simulink model "usb01deneme_hazin"  (R2023a)
settings: Solver=ode5  StartTime=0.0  StopTime=inf  RelTol=1e-3
InitFcn:
  | usbsetup
values from neighbouring files (symbols this model uses):
  K = 1    [usbsetup.m]
  T = Ts    (= 0.01)    [usbsetup.m]
  Td = 0.01    [usbsetup.m]
  Ti = 1    [usbsetup.m]
  Ts_rec = 0.5e-3    (= 0.0005)    [usbsetup.m]
  Ts_send = 0.5e-3    (= 0.0005)    [usbsetup.m]
undefined symbols (not defined in the file or in its folder): Dz, Kd, Serial_Port, Standard_Devices, z0, zp
libraries: sldrtlib x18, dsparch4 x9, slpidlib x1
settings Model: SimulationMode=external  Creator=halil  LastModifiedBy=halil
settings DataIOCC: ReturnWorkspaceOutputs=off
settings DebuggingCC: ParameterPrecisionLossMsg=none
settings HardwareCC: ProdBitPerLong=64  ProdHWDeviceType=Intel->x86-64 (Linux 64)
settings RTWCC: Description=Simulink Desktop Real-Time  SystemTargetFile=sldrt.tlc  TemplateMakefile=sldrt.tmf  RTWCompilerOptimization=on
settings CodeAppCC: MaxIdLength=95
settings SimulinkDesktopRealTimeCC: TargetLibSuffix=_sldrt.a  TargetPreCompLibLocation=C:\Program Files\MATLAB\R2023a\toolbox\sldrt\lib\win64

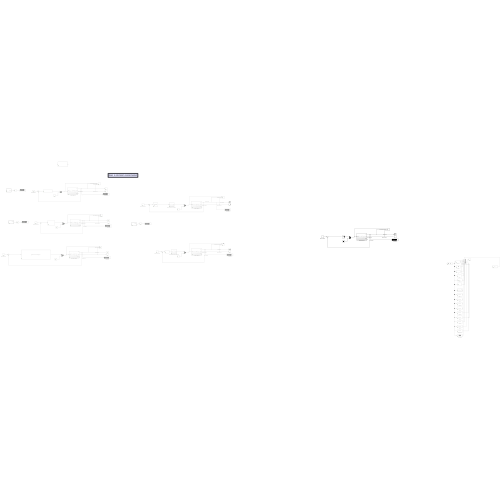
[thumbnail: Simulink's stored preview of the top-level diagram]
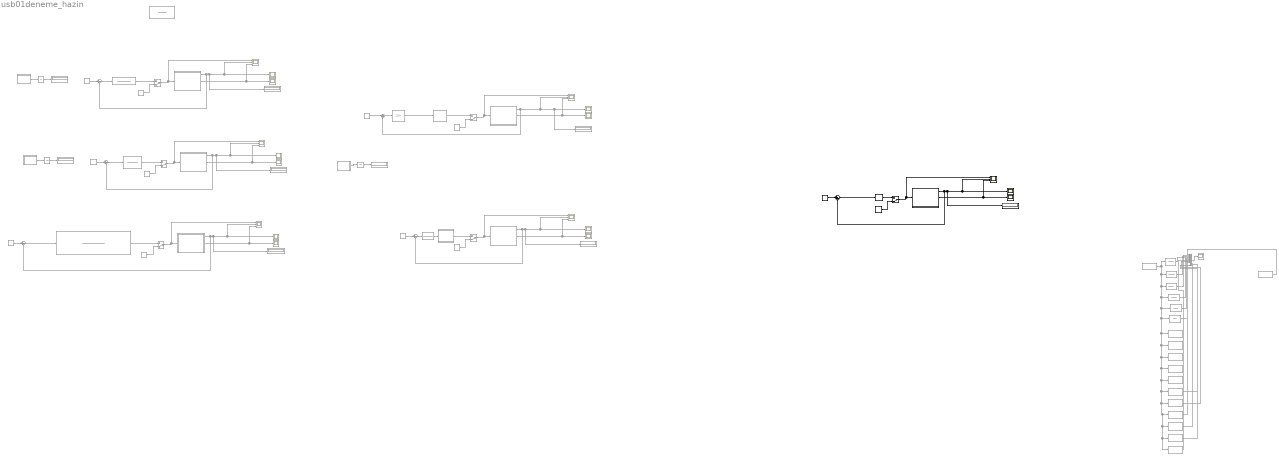
== system usb01deneme_hazin ==
  note: Bazı z-domain çalışmaları
  100fc : TransferFcn  Commented=on  Numerator=[100 0]  Denominator=[1 100]
  1fc : TransferFcn  Commented=on  Numerator=[1 0]  Denominator=[1 1]
  25fc : TransferFcn  Commented=on  Numerator=[25 0]  Denominator=[1 25]
  50fc : TransferFcn  Commented=on  Numerator=[50 0]  Denominator=[1 50]
  5fc : TransferFcn  Commented=on  Numerator=[5 0]  Denominator=[1 5]
  75fc : TransferFcn  Commented=on  Numerator=[75 0]  Denominator=[1 75]
  Angle(deg) : Display
  Angle(deg){1..4,6} (5 alike) : Display  Commented=on
  BugüzelMi? : dsparch4/Biquad Filter  Tag=BlockMethodSubSystem  Commented=on  FilterSource=Dialog parameters  CoeffSource=Specify via dialog  FilterObject=BQF  IIRFiltStruct=Direct form II  BiQuadCoeffs=[1 -1 0 1 -0.999373367998741768 0]  ScaleValues=[0.999686683999370884;1]  IC=0  ICnum=0  ICden=0  a0Flag=Warning  optimizeScaleValues=on  ScaleValueMode=Specify via input port (g)  InputProcessing=Columns as channels (frame based)  roundingMode=Floor  overflowMode=off  scaleValueFracLength=14  denProdOutputFracLength=30  denAccumFracLength=30  secondMemoryFracLength=15
  Constant : Constant  Value=0
  Constant{1..4,6} (5 alike) : Constant  Commented=on  Value=0
  DC Motor Sistemi : Subsystem
  DC Motor Sistemi1 : Subsystem  Commented=on
  DC Motor Sistemi2 : Subsystem  Commented=on
  DC Motor Sistemi3 : Subsystem  Commented=on
  DC Motor Sistemi4 : Subsystem  Commented=on
  DC Motor Sistemi6 : Subsystem  Commented=on
  Data Type Conversion : DataTypeConversion  Commented=on  OutDataTypeStr=double  SaturateOnIntegerOverflow=off  RndMeth=Floor
  Data Type Conversion1 : DataTypeConversion  Commented=on  OutDataTypeStr=double  SaturateOnIntegerOverflow=off  RndMeth=Floor
  Discrete Transfer Fcn : DiscreteTransferFcn  Commented=on  Numerator=[2 -0.2]  Denominator=[1 (1-0.2)]
  Discrete Transfer Fcn1 : DiscreteTransferFcn  Commented=on  Numerator=[(Kd) (-Kd*z0)]  Denominator=[1 (-zp)]  SampleTime=T
  Discrete Transfer Fcn2 : DiscreteTransferFcn  Commented=on  Numerator=[37.5 -37.2]  Denominator=[1 -0.7]  SampleTime=T
  Discrete Transfer Fcn4 : DiscreteTransferFcn  Commented=on  Numerator=[Dz.numerator{1,1}]  Denominator=[Dz.denominator{1,1}]  SampleTime=T
  Display : Display  Commented=on
  Display1 : Display  Commented=on
  Display2 : Display  Commented=on
  Filter : dsparch4/Biquad Filter  Tag=BlockMethodSubSystem  Commented=on  FilterSource=Dialog parameters  CoeffSource=Specify via dialog  FilterObject=BQF  IIRFiltStruct=Direct form II  BiQuadCoeffs=[1 -2 1 1 1.63889042744449531 0.78299941352519975;1 -2 1 1 1.39413928992720804 0.516727106758841592;1 -1 0 1 0.659452728771293573 0]  ScaleValues=[0.0360272465201760816;0.0306469542079083335;0.170273635614353186;1]  IC=0  ICnum=0  ICden=0  a0Flag=Warning  optimizeScaleValues=on  ScaleValueMode=Specify via input port (g)  InputProcessing=Columns as channels (frame based)  roundingMode=Floor  overflowMode=off  scaleValueFracLength=14  denProdOutputFracLength=30  denAccumFracLength=30  secondMemoryFracLength=15
  Filter1 : dsparch4/Biquad Filter  Tag=BlockMethodSubSystem  Commented=on  FilterSource=Dialog parameters  CoeffSource=Specify via dialog  FilterObject=BQF  IIRFiltStruct=Direct form II  BiQuadCoeffs=[1 -2 1 1 -0.751668315831577671 0.502252814025592853;1 -2 1 1 -0.555983969636365316 0.111166275533815195]  ScaleValues=[0.563480282464292603;0.416787561292545128;1]  IC=0  ICnum=0  ICden=0  a0Flag=Warning  optimizeScaleValues=on  ScaleValueMode=Specify via input port (g)  InputProcessing=Columns as channels (frame based)  roundingMode=Floor  overflowMode=off  scaleValueFracLength=14  denProdOutputFracLength=30  denAccumFracLength=30  secondMemoryFracLength=15
  Filter2 : dsparch4/Biquad Filter  Tag=BlockMethodSubSystem  Commented=on  FilterSource=Dialog parameters  CoeffSource=Specify via dialog  FilterObject=BQF  IIRFiltStruct=Direct form II  BiQuadCoeffs=[1 -2 1 1 -1.7220160678191494 0.756195048099618239]  ScaleValues=[0.869552778979691854;1]  IC=0  ICnum=0  ICden=0  a0Flag=Warning  optimizeScaleValues=on  ScaleValueMode=Specify via input port (g)  InputProcessing=Columns as channels (frame based)  roundingMode=Floor  overflowMode=off  scaleValueFracLength=14  denProdOutputFracLength=30  denAccumFracLength=30  secondMemoryFracLength=15
  Filter3 : dsparch4/Biquad Filter  Tag=BlockMethodSubSystem  Commented=on  FilterSource=Dialog parameters  CoeffSource=Specify via dialog  FilterObject=BQF  IIRFiltStruct=Direct form II  BiQuadCoeffs=[1 -2 1 1 -1.97197387617265707 0.972361217649310716]  ScaleValues=[0.986083773455491919;1]  IC=0  ICnum=0  ICden=0  a0Flag=Warning  optimizeScaleValues=on  ScaleValueMode=Specify via input port (g)  InputProcessing=Columns as channels (frame based)  roundingMode=Floor  overflowMode=off  scaleValueFracLength=14  denProdOutputFracLength=30  denAccumFracLength=30  secondMemoryFracLength=15
  Filter4 : dsparch4/Biquad Filter  Tag=BlockMethodSubSystem  Commented=on  FilterSource=Dialog parameters  CoeffSource=Specify via dialog  FilterObject=BQF  IIRFiltStruct=Direct form II  BiQuadCoeffs=[1 -1 0 1 -0.993767790272316875 0]  ScaleValues=[0.996883895136158382;1]  IC=0  ICnum=0  ICden=0  a0Flag=Warning  optimizeScaleValues=on  ScaleValueMode=Specify via input port (g)  InputProcessing=Columns as channels (frame based)  roundingMode=Floor  overflowMode=off  scaleValueFracLength=14  denProdOutputFracLength=30  denAccumFracLength=30  secondMemoryFracLength=15
  Filter5 : dsparch4/Biquad Filter  Tag=BlockMethodSubSystem  Commented=on  FilterSource=Dialog parameters  CoeffSource=Specify via dialog  FilterObject=BQF  IIRFiltStruct=Direct form II  BiQuadCoeffs=[1 -1 0 1 -0.981326377391473437 0]  ScaleValues=[0.990663188695736663;1]  IC=0  ICnum=0  ICden=0  a0Flag=Warning  optimizeScaleValues=on  ScaleValueMode=Specify via input port (g)  InputProcessing=Columns as channels (frame based)  roundingMode=Floor  overflowMode=off  scaleValueFracLength=14  denProdOutputFracLength=30  denAccumFracLength=30  secondMemoryFracLength=15
  Filter6 : dsparch4/Biquad Filter  Tag=BlockMethodSubSystem  Commented=on  FilterSource=Dialog parameters  CoeffSource=Specify via dialog  FilterObject=BQF  IIRFiltStruct=Direct form II  BiQuadCoeffs=[1 -1 0 1 -0.998456046873542391 0]  ScaleValues=[0.999228023436771196;1]  IC=0  ICnum=0  ICden=0  a0Flag=Warning  optimizeScaleValues=on  ScaleValueMode=Specify via input port (g)  InputProcessing=Columns as channels (frame based)  roundingMode=Floor  overflowMode=off  scaleValueFracLength=14  denProdOutputFracLength=30  denAccumFracLength=30  secondMemoryFracLength=15
  Filter7 : dsparch4/Biquad Filter  Tag=BlockMethodSubSystem  Commented=on  FilterSource=Dialog parameters  CoeffSource=Specify via dialog  FilterObject=BQF  IIRFiltStruct=Direct form II  BiQuadCoeffs=[1 -1 0 1 -0.999227725423996294 0]  ScaleValues=[0.999613862711998147;1]  IC=0  ICnum=0  ICden=0  a0Flag=Warning  optimizeScaleValues=on  ScaleValueMode=Specify via input port (g)  InputProcessing=Columns as channels (frame based)  roundingMode=Floor  overflowMode=off  scaleValueFracLength=14  denProdOutputFracLength=30  denAccumFracLength=30  secondMemoryFracLength=15
  Integrator : Integrator  Commented=on
  Integrator1 : Integrator  Commented=on
  Integrator2 : Integrator  Commented=on
  MATLAB Function : MATLAB Function  Commented=on  TreatAsAtomicUnit=on
  MATLAB Function1 : MATLAB Function  Commented=on  TreatAsAtomicUnit=on
  MATLAB Function2 : MATLAB Function  Commented=on  TreatAsAtomicUnit=on
  Manual Switch : ManualSwitch  CurrentSetting=0
  Manual Switch{1..4,6} (5 alike) : ManualSwitch  Commented=on  CurrentSetting=0
  Mux : Mux  Commented=on  Inputs=13
  PID Controller1 : slpidlib/PID Controller  Controller=PID  Form=Ideal  TimeDomain=Continuous-time  UseExternalTs=off  SampleTime=-1  IntegratorMethod=Forward Euler  FilterMethod=Forward Euler  ControllerParametersSource=internal  P=1  I=1  UseKiTs=off  D=0.01  N=100  UseFilter=on  TunerSelectOption=Transfer Function Based (PID Tuner App)  InitialConditionSource=internal  InitialConditionForIntegrator=0  InitialConditionForFilter=0  DifferentiatorICPrevScaledInput=0  ExternalReset=none  TrackingMode=off  Kt=1  LimitOutput=on  SatLimitsSource=internal  UpperSaturationLimit=6  LowerSaturationLimit=-6  LinearizeAsGain=off  AntiWindupMode=none  Kb=1  LimitIntegrator=off  UpperIntegratorSaturationLimit=inf  LowerIntegratorSaturationLimit=-inf  POutMin=[]  POutMax=[]  IOutMin=[]  IOutMax=[]  DOutMin=[]  DOutMax=[]  NOutMin=[]  NOutMax=[]  SumOutMin=[]  SumOutMax=[]  SaturationOutMin=[]  SaturationOutMax=[]  PParamMin=[]  PParamMax=[]  IParamMin=[]  IParamMax=[]  DParamMin=[]  DParamMax=[]  NParamMin=[]  NParamMax=[]  KbParamMin=[]  KbParamMax=[]  KtParamMin=[]  KtParamMax=[]  KbOutMin=[]  KbOutMax=[]  KtOutMin=[]  KtOutMax=[]  IntegratorOutMin=[]  IntegratorOutMax=[]  FilterOutMin=[]  FilterOutMax=[]  SumI1OutMin=[]  SumI1OutMax=[]  SumI2OutMin=[]  SumI2OutMax=[]  SumI3OutMin=[]  SumI3OutMax=[]  SumI4OutMin=[]  SumI4OutMax=[]  SumDOutMin=[]  SumDOutMax=[]  DifferentiatorOutMin=[]  DifferentiatorOutMax=[]  FilterDiffOutCoefMin=[]  FilterDiffOutCoefMax=[]  ReciprocalOutMin=[]  ReciprocalOutMax=[]  SumDenOutMin=[]  SumDenOutMax=[]  SumNumOutMin=[]  SumNumOutMax=[]  DivideOutMin=[]  DivideOutMax=[]  UdiffTsProdOutMin=[]  UdiffTsProdOutMax=[]  NTsProdOutMin=[]  NTsProdOutMax=[]  UintegralTsProdOutMin=[]  UintegralTsProdOutMax=[]  UngainTsProdOutMin=[]  UngainTsProdOutMax=[]  ClampingZeroOutDataTypeStr=Inherit: Inherit via back propagation  ClampingZeroOutMin=[]  ClampingZeroOutMax=[]  FilterDenConstantOutDataTypeStr=Inherit: Inherit via back propagation  FilterDenConstantOutMin=[]  FilterDenConstantOutMax=[]  PCopyOutDataTypeStr=Inherit: Inherit via back propagation  PCopyOutMin=[]  PCopyOutMax=[]  NCopyOutDataTypeStr=Inherit: Inherit via back propagation  NCopyOutMin=[]  NCopyOutMax=[]  IntegratorContinuousStateAttributes=''  IntegratorStateMustResolveToSignalObject=off  IntegratorRTWStateStorageClass=Auto  FilterContinuousStateAttributes=''  FilterStateMustResolveToSignalObject=off  FilterRTWStateStorageClass=Auto  ParallelPVariant=Passthrough  IdealPVariant=InternalParameters  IVariant=InternalParameters  DVariant=InternalParameters  IntegratorVariant=Continuous  SatVariant=Enabled  AWVariant=Passthrough  PCopyVariant=Disabled  TRVariant=Disabled  FdbkBlocksVariant=Forward  IdealPFdbkVariant=Disabled  SatFdbkVariant=Disabled  DerivativeFilterVariant=ContFilter  NVariant=InternalParameters  NCopyVariant=Disabled  FilterICVariant=InternalICsFilter  IntegratorICVariant=InternalICs  ExternalResetVariant=Disabled  TRSumVariant=Passthrough  SumFdbkVariant=Disabled  SumVariant=Sum_PID  TsampFilterVariant=InternalTs  TsampNgainVariant=Passthrough  TsampIntegralVariant=Disabled_SignalSpec  ExternalSaturationOutDataTypeStr=Inherit: Same as second input
  PID(frequence domain emulation) : Subsystem  Commented=on
  PID(time domain emulation) : Subsystem  Commented=on
  Scope{,4,6,8..9,11..12,14..15,20..21} (11 alike) : Scope  Commented=on
  Scope1 : Scope  NumInputPorts=3
  Scope{2,7,10,13,19} (5 alike) : Scope  Commented=on  NumInputPorts=3
  Scope3 : Scope
  Scope5 : Scope
  Sum : Sum  Inputs=|+-
  Sum{1..4,6} (5 alike) : Sum  Commented=on  Inputs=|+-
  Transfer Fcn1 : TransferFcn  Commented=on  Numerator=[90/2.1]  Denominator=[0.2/4 1]
  Zero-Order Hold : ZeroOrderHold  Commented=on  SampleTime=T
  differentiFilter : DiscreteFir  Tag=BlockMethodSubSystem  Commented=on  Coefficients=[0.10162245249798578 0.462115751014000098 -0.462115751014000098 -0.10162245249798578]  InputProcessing=Columns as channels (frame based)
  numericd1 : Subsystem  Tag=BlockMethodSubSystem  Commented=on
  setPoint(degree) : Constant  Value=100
  setPoint(degree)1 : Constant  Commented=on  Value=0
  setPoint(degree)2 : Constant  Commented=on  Value=100
  setPoint(degree)3 : Constant  Commented=on  Value=100
  setPoint(degree)4 : Constant  Commented=on  Value=100
  setPoint(degree)6 : Constant  Commented=on  Value=0
  wires:
  DC Motor Sistemi/1(Açı) -> Sum/2, Scope1/2, Scope3/1, Angle(deg)/1  "Angle(degree)"
  Sum/1 -> PID Controller1/1
  50fc/1 -> Mux/4  "dq"
  Mux/1 -> Scope/1
  Data Type Conversion/1 -> differentiFilter/1, BugüzelMi?/1, Filter7/1, Filter6/1, Filter5/1, Filter4/1, Filter3/1, Filter2/1, Filter1/1, Filter/1, numericd1/1(In), 1fc/1, 5fc/1, 25fc/1, 75fc/1, 100fc/1, 50fc/1
  Constant/1 -> Manual Switch/2
  Manual Switch/1 -> Scope1/1, DC Motor Sistemi/1(Voltaj)  "control signal(u)(Voltage)"
  Data Type Conversion1/1 -> Mux/1
  100fc/1 -> Mux/3
  75fc/1 -> Mux/2
  25fc/1 -> Mux/5
  5fc/1 -> Mux/6
  Filter4/1 -> Mux/13
  Filter5/1 -> Mux/9
  Filter6/1 -> Mux/10
  Filter7/1 -> Mux/11
  BugüzelMi?/1 -> Mux/12
  differentiFilter/1 -> Mux/8
  DC Motor Sistemi/2(Hız) -> Scope1/3, Scope5/1  "filteredSpeed(1/s)"
  1fc/1 -> Mux/7
  PID Controller1/1 -> Manual Switch/1
  setPoint(degree)/1 -> Sum/1
  Manual Switch1/1 -> Scope2/1, DC Motor Sistemi1/1(Voltaj)  "control signal(u)(Voltage)"
  DC Motor Sistemi1/2(Hız) -> Scope2/3, Scope6/1  "filteredSpeed(1/s)"
  PID(time domain emulation)/1(u[k]) -> Manual Switch1/1
  Constant1/1 -> Manual Switch1/2
  DC Motor Sistemi1/1(Açı) -> Scope2/2, Angle(deg)1/1, Scope4/1, Sum1/2  "Angle(degree)"
  setPoint(degree)1/1 -> Sum1/1
  Sum1/1 -> Zero-Order Hold/1
  Zero-Order Hold/1 -> PID(time domain emulation)/1(e[k])
  setPoint(degree)2/1 -> Sum3/1
  Manual Switch2/1 -> Scope7/1, DC Motor Sistemi2/1(Voltaj)  "control signal(u)(Voltage)"
  DC Motor Sistemi2/2(Hız) -> Scope7/3, Scope9/1  "filteredSpeed(1/s)"
  PID(frequence domain emulation)/1(u(t)) -> Manual Switch2/1
  Constant2/1 -> Manual Switch2/2
  DC Motor Sistemi2/1(Açı) -> Sum3/2, Scope7/2, Scope8/1, Angle(deg)2/1  "Angle(degree)"
  Discrete Transfer Fcn/1 -> PID(frequence domain emulation)/1(e(t))
  Sum3/1 -> Discrete Transfer Fcn/1
  DC Motor Sistemi3/2(Hız) -> Scope10/3, Scope12/1  "filteredSpeed(1/s)"
  Constant3/1 -> Manual Switch3/2
  DC Motor Sistemi3/1(Açı) -> Sum2/2, Scope10/2, Scope11/1, Angle(deg)3/1  "Angle(degree)"
  setPoint(degree)3/1 -> Sum2/1
  Manual Switch3/1 -> Scope10/1, DC Motor Sistemi3/1(Voltaj)  "control signal(u)(Voltage)"
  Sum2/1 -> Discrete Transfer Fcn1/1
  Discrete Transfer Fcn1/1 -> Manual Switch3/1
  MATLAB Function/1(norme) -> Integrator/1
  Integrator/1 -> Display/1
  Integrator1/1 -> Display1/1
  MATLAB Function1/1(norme) -> Integrator1/1
  Constant4/1 -> Manual Switch4/2
  DC Motor Sistemi4/2(Hız) -> Scope13/3, Scope15/1  "filteredSpeed(1/s)"
  Manual Switch4/1 -> Scope13/1, DC Motor Sistemi4/1(Voltaj)  "control signal(u)(Voltage)"
  DC Motor Sistemi4/1(Açı) -> Sum4/2, Scope13/2, Scope14/1, Angle(deg)4/1  "Angle(degree)"
  Discrete Transfer Fcn2/1 -> Manual Switch4/1
  setPoint(degree)4/1 -> Sum4/1
  Sum4/1 -> Discrete Transfer Fcn2/1
  MATLAB Function2/1(norme) -> Integrator2/1
  Integrator2/1 -> Display2/1
  Sum6/1 -> Discrete Transfer Fcn4/1
  setPoint(degree)6/1 -> Sum6/1
  Discrete Transfer Fcn4/1 -> Manual Switch6/1
  Manual Switch6/1 -> Scope19/1, DC Motor Sistemi6/1(Voltaj)  "control signal(u)(Voltage)"
  Constant6/1 -> Manual Switch6/2
  DC Motor Sistemi6/2(Hız) -> Scope19/3, Scope21/1  "filteredSpeed(1/s)"
  DC Motor Sistemi6/1(Açı) -> Sum6/2, Scope19/2, Scope20/1, Angle(deg)6/1  "Angle(degree)"

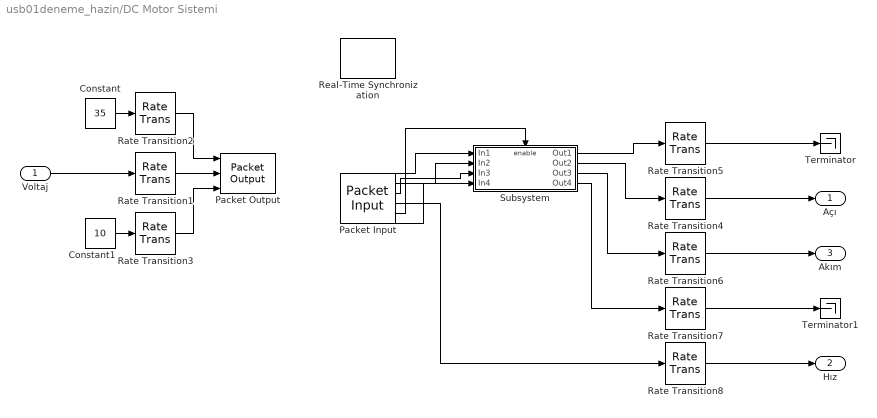
== system usb01deneme_hazin/DC Motor Sistemi ==
  Voltaj : Inport
  Constant : Constant  Value=35
  Constant1 : Constant  Value=10
  Packet Input : sldrtlib/Packet Input  SampleTime=Ts_rec  MaxMissedTicks=1000  ShowMissedTicks=off  YieldWhenWaiting=off  DrvName=Standard_Devices/Serial_Port  DrvAddress=4  DrvOptions=[9600 8 0 0 0 0 0 0]  PacketSize=14  DataTypes={'uint8','single','single','single','uint8'}  ShowReady=on  ShowError=off  PacketID=1  ByteOrder=1  ShowTimestamp=off
      settings: AttributesFormatString=Serial Port [4]
  Packet Output : sldrtlib/Packet Output  SampleTime=Ts_send  MaxMissedTicks=1000  ShowMissedTicks=off  YieldWhenWaiting=off  DrvName=Standard_Devices/Serial_Port  DrvAddress=4  DrvOptions=[9600 8 0 0 0 0 0 0]  PacketSize=6  DataTypes={'uint8','single','uint8'}  ShowReady=off  ShowError=off  PacketID=1  ByteOrder=1  InitialValue=[]  FinalValue=[]
      settings: AttributesFormatString=Serial Port [4]
  Rate Transition1 : RateTransition  OutPortSampleTime=Ts_send
  Rate Transition2 : RateTransition  OutPortSampleTime=Ts_send
  Rate Transition3 : RateTransition  OutPortSampleTime=Ts_send
  Rate Transition{4..8} (5 alike) : RateTransition  OutPortSampleTime=Ts_algo
  Real-Time Synchronization : sldrtlib/Real-Time Synchronization  SampleTime=Ts_rec  MaxMissedTicks=1000  ShowMissedTicks=off  YieldWhenWaiting=off
  Subsystem : Subsystem
  Terminator : Terminator
  Terminator1 : Terminator
  Açı : Outport
  Hız : Outport  Port=2
  Akım : Outport  Port=3
  wires:
  Rate Transition3/1 -> Packet Output/3
  Rate Transition1/1 -> Packet Output/2
  Subsystem/1(Out1) -> Rate Transition5/1
  Packet Input/2 -> Subsystem/2(In2)
  Rate Transition2/1 -> Packet Output/1
  Packet Input/3 -> Subsystem/3(In3)
  Subsystem/3(Out3) -> Rate Transition6/1
  Subsystem/4(Out4) -> Rate Transition7/1
  Packet Input/1 -> Subsystem/1(In1)
  Packet Input/5 -> Subsystem/Enable
  Subsystem/2(Out2) -> Rate Transition4/1
  Rate Transition4/1 -> Açı/1
  Voltaj/1 -> Rate Transition1/1
  Constant/1 -> Rate Transition2/1
  Rate Transition7/1 -> Terminator1/1
  Constant1/1 -> Rate Transition3/1
  Rate Transition5/1 -> Terminator/1
  Packet Input/4 -> Rate Transition8/1
  Rate Transition8/1 -> Hız/1
  Packet Input/6 -> Subsystem/4(In4)
  Rate Transition6/1 -> Akım/1

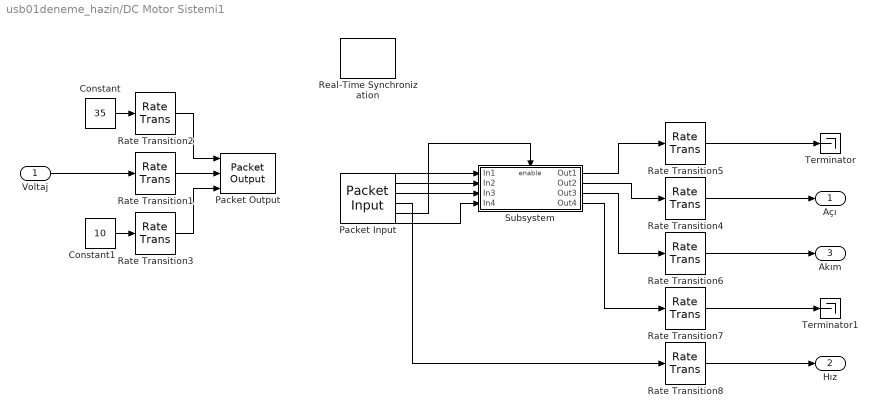
== system usb01deneme_hazin/DC Motor Sistemi1 ==
  Voltaj : Inport
  Constant : Constant  Value=35
  Constant1 : Constant  Value=10
  Packet Input : sldrtlib/Packet Input  SampleTime=Ts_rec  MaxMissedTicks=1000  ShowMissedTicks=off  YieldWhenWaiting=off  DrvName=Standard_Devices/Serial_Port  DrvAddress=4  DrvOptions=[9600 8 0 0 0 0 0 0]  PacketSize=14  DataTypes={'uint8','single','single','single','uint8'}  ShowReady=on  ShowError=off  PacketID=1  ByteOrder=1  ShowTimestamp=off
      settings: AttributesFormatString=Serial Port [4]
  Packet Output : sldrtlib/Packet Output  SampleTime=Ts_send  MaxMissedTicks=1000  ShowMissedTicks=off  YieldWhenWaiting=off  DrvName=Standard_Devices/Serial_Port  DrvAddress=4  DrvOptions=[9600 8 0 0 0 0 0 0]  PacketSize=6  DataTypes={'uint8','single','uint8'}  ShowReady=off  ShowError=off  PacketID=1  ByteOrder=1  InitialValue=[]  FinalValue=[]
      settings: AttributesFormatString=Serial Port [4]
  Rate Transition1 : RateTransition  OutPortSampleTime=Ts_send
  Rate Transition2 : RateTransition  OutPortSampleTime=Ts_send
  Rate Transition3 : RateTransition  OutPortSampleTime=Ts_send
  Rate Transition{4..8} (5 alike) : RateTransition  OutPortSampleTime=Ts_algo
  Real-Time Synchronization : sldrtlib/Real-Time Synchronization  SampleTime=Ts_rec  MaxMissedTicks=1000  ShowMissedTicks=off  YieldWhenWaiting=off
  Subsystem : Subsystem
  Terminator : Terminator
  Terminator1 : Terminator
  Açı : Outport
  Hız : Outport  Port=2
  Akım : Outport  Port=3
  wires:
  Rate Transition3/1 -> Packet Output/3
  Rate Transition1/1 -> Packet Output/2
  Subsystem/1(Out1) -> Rate Transition5/1
  Packet Input/2 -> Subsystem/2(In2)
  Rate Transition2/1 -> Packet Output/1
  Packet Input/3 -> Subsystem/3(In3)
  Subsystem/3(Out3) -> Rate Transition6/1
  Subsystem/4(Out4) -> Rate Transition7/1
  Packet Input/1 -> Subsystem/1(In1)
  Packet Input/5 -> Subsystem/Enable
  Subsystem/2(Out2) -> Rate Transition4/1
  Rate Transition4/1 -> Açı/1
  Voltaj/1 -> Rate Transition1/1
  Constant/1 -> Rate Transition2/1
  Rate Transition7/1 -> Terminator1/1
  Constant1/1 -> Rate Transition3/1
  Rate Transition5/1 -> Terminator/1
  Packet Input/4 -> Rate Transition8/1
  Rate Transition8/1 -> Hız/1
  Packet Input/6 -> Subsystem/4(In4)
  Rate Transition6/1 -> Akım/1

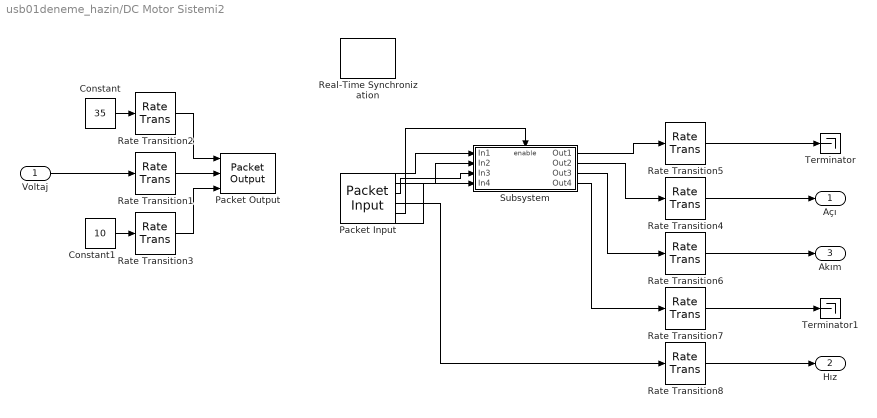
== system usb01deneme_hazin/DC Motor Sistemi2 ==
  Voltaj : Inport
  Constant : Constant  Value=35
  Constant1 : Constant  Value=10
  Packet Input : sldrtlib/Packet Input  SampleTime=Ts_rec  MaxMissedTicks=1000  ShowMissedTicks=off  YieldWhenWaiting=off  DrvName=Standard_Devices/Serial_Port  DrvAddress=4  DrvOptions=[9600 8 0 0 0 0 0 0]  PacketSize=14  DataTypes={'uint8','single','single','single','uint8'}  ShowReady=on  ShowError=off  PacketID=1  ByteOrder=1  ShowTimestamp=off
      settings: AttributesFormatString=Serial Port [4]
  Packet Output : sldrtlib/Packet Output  SampleTime=Ts_send  MaxMissedTicks=1000  ShowMissedTicks=off  YieldWhenWaiting=off  DrvName=Standard_Devices/Serial_Port  DrvAddress=4  DrvOptions=[9600 8 0 0 0 0 0 0]  PacketSize=6  DataTypes={'uint8','single','uint8'}  ShowReady=off  ShowError=off  PacketID=1  ByteOrder=1  InitialValue=[]  FinalValue=[]
      settings: AttributesFormatString=Serial Port [4]
  Rate Transition1 : RateTransition  OutPortSampleTime=Ts_send
  Rate Transition2 : RateTransition  OutPortSampleTime=Ts_send
  Rate Transition3 : RateTransition  OutPortSampleTime=Ts_send
  Rate Transition{4..8} (5 alike) : RateTransition  OutPortSampleTime=Ts_algo
  Real-Time Synchronization : sldrtlib/Real-Time Synchronization  SampleTime=Ts_rec  MaxMissedTicks=1000  ShowMissedTicks=off  YieldWhenWaiting=off
  Subsystem : Subsystem
  Terminator : Terminator
  Terminator1 : Terminator
  Açı : Outport
  Hız : Outport  Port=2
  Akım : Outport  Port=3
  wires:
  Rate Transition3/1 -> Packet Output/3
  Rate Transition1/1 -> Packet Output/2
  Subsystem/1(Out1) -> Rate Transition5/1
  Packet Input/2 -> Subsystem/2(In2)
  Rate Transition2/1 -> Packet Output/1
  Packet Input/3 -> Subsystem/3(In3)
  Subsystem/3(Out3) -> Rate Transition6/1
  Subsystem/4(Out4) -> Rate Transition7/1
  Packet Input/1 -> Subsystem/1(In1)
  Packet Input/5 -> Subsystem/Enable
  Subsystem/2(Out2) -> Rate Transition4/1
  Rate Transition4/1 -> Açı/1
  Voltaj/1 -> Rate Transition1/1
  Constant/1 -> Rate Transition2/1
  Rate Transition7/1 -> Terminator1/1
  Constant1/1 -> Rate Transition3/1
  Rate Transition5/1 -> Terminator/1
  Packet Input/4 -> Rate Transition8/1
  Rate Transition8/1 -> Hız/1
  Packet Input/6 -> Subsystem/4(In4)
  Rate Transition6/1 -> Akım/1

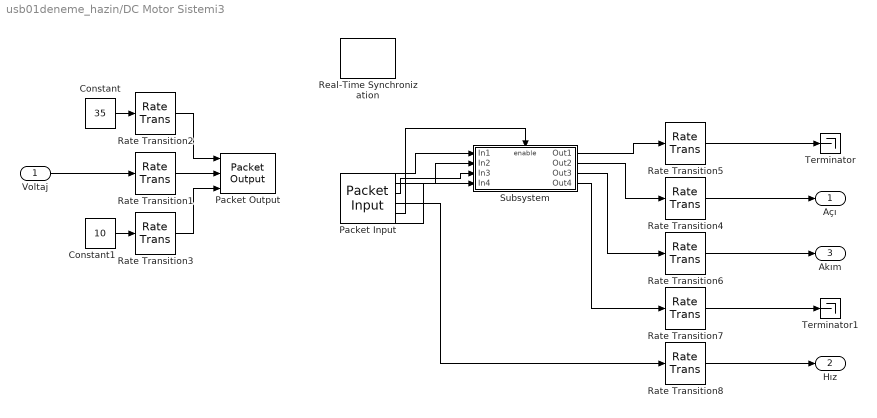
== system usb01deneme_hazin/DC Motor Sistemi3 ==
  Voltaj : Inport
  Constant : Constant  Value=35
  Constant1 : Constant  Value=10
  Packet Input : sldrtlib/Packet Input  SampleTime=Ts_rec  MaxMissedTicks=1000  ShowMissedTicks=off  YieldWhenWaiting=off  DrvName=Standard_Devices/Serial_Port  DrvAddress=4  DrvOptions=[9600 8 0 0 0 0 0 0]  PacketSize=14  DataTypes={'uint8','single','single','single','uint8'}  ShowReady=on  ShowError=off  PacketID=1  ByteOrder=1  ShowTimestamp=off
      settings: AttributesFormatString=Serial Port [4]
  Packet Output : sldrtlib/Packet Output  SampleTime=Ts_send  MaxMissedTicks=1000  ShowMissedTicks=off  YieldWhenWaiting=off  DrvName=Standard_Devices/Serial_Port  DrvAddress=4  DrvOptions=[9600 8 0 0 0 0 0 0]  PacketSize=6  DataTypes={'uint8','single','uint8'}  ShowReady=off  ShowError=off  PacketID=1  ByteOrder=1  InitialValue=[]  FinalValue=[]
      settings: AttributesFormatString=Serial Port [4]
  Rate Transition1 : RateTransition  OutPortSampleTime=Ts_send
  Rate Transition2 : RateTransition  OutPortSampleTime=Ts_send
  Rate Transition3 : RateTransition  OutPortSampleTime=Ts_send
  Rate Transition{4..8} (5 alike) : RateTransition  OutPortSampleTime=Ts_algo
  Real-Time Synchronization : sldrtlib/Real-Time Synchronization  SampleTime=Ts_rec  MaxMissedTicks=1000  ShowMissedTicks=off  YieldWhenWaiting=off
  Subsystem : Subsystem
  Terminator : Terminator
  Terminator1 : Terminator
  Açı : Outport
  Hız : Outport  Port=2
  Akım : Outport  Port=3
  wires:
  Rate Transition3/1 -> Packet Output/3
  Rate Transition1/1 -> Packet Output/2
  Subsystem/1(Out1) -> Rate Transition5/1
  Packet Input/2 -> Subsystem/2(In2)
  Rate Transition2/1 -> Packet Output/1
  Packet Input/3 -> Subsystem/3(In3)
  Subsystem/3(Out3) -> Rate Transition6/1
  Subsystem/4(Out4) -> Rate Transition7/1
  Packet Input/1 -> Subsystem/1(In1)
  Packet Input/5 -> Subsystem/Enable
  Subsystem/2(Out2) -> Rate Transition4/1
  Rate Transition4/1 -> Açı/1
  Voltaj/1 -> Rate Transition1/1
  Constant/1 -> Rate Transition2/1
  Rate Transition7/1 -> Terminator1/1
  Constant1/1 -> Rate Transition3/1
  Rate Transition5/1 -> Terminator/1
  Packet Input/4 -> Rate Transition8/1
  Rate Transition8/1 -> Hız/1
  Packet Input/6 -> Subsystem/4(In4)
  Rate Transition6/1 -> Akım/1

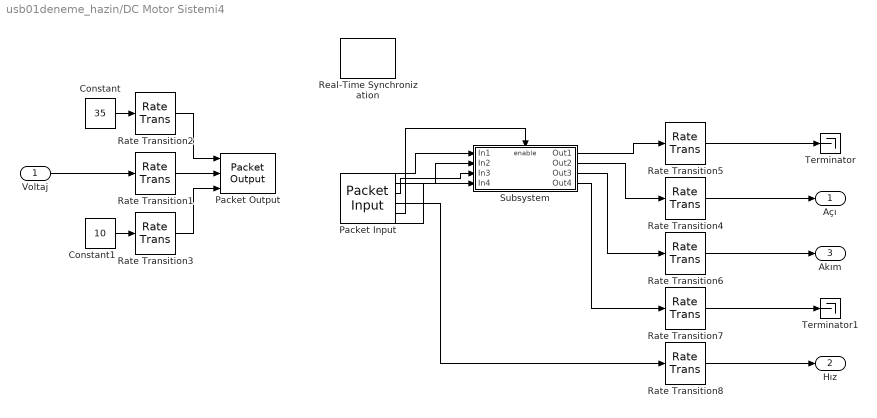
== system usb01deneme_hazin/DC Motor Sistemi4 ==
  Voltaj : Inport
  Constant : Constant  Value=35
  Constant1 : Constant  Value=10
  Packet Input : sldrtlib/Packet Input  SampleTime=Ts_rec  MaxMissedTicks=1000  ShowMissedTicks=off  YieldWhenWaiting=off  DrvName=Standard_Devices/Serial_Port  DrvAddress=4  DrvOptions=[9600 8 0 0 0 0 0 0]  PacketSize=14  DataTypes={'uint8','single','single','single','uint8'}  ShowReady=on  ShowError=off  PacketID=1  ByteOrder=1  ShowTimestamp=off
      settings: AttributesFormatString=Serial Port [4]
  Packet Output : sldrtlib/Packet Output  SampleTime=Ts_send  MaxMissedTicks=1000  ShowMissedTicks=off  YieldWhenWaiting=off  DrvName=Standard_Devices/Serial_Port  DrvAddress=4  DrvOptions=[9600 8 0 0 0 0 0 0]  PacketSize=6  DataTypes={'uint8','single','uint8'}  ShowReady=off  ShowError=off  PacketID=1  ByteOrder=1  InitialValue=[]  FinalValue=[]
      settings: AttributesFormatString=Serial Port [4]
  Rate Transition1 : RateTransition  OutPortSampleTime=Ts_send
  Rate Transition2 : RateTransition  OutPortSampleTime=Ts_send
  Rate Transition3 : RateTransition  OutPortSampleTime=Ts_send
  Rate Transition{4..8} (5 alike) : RateTransition  OutPortSampleTime=Ts_algo
  Real-Time Synchronization : sldrtlib/Real-Time Synchronization  SampleTime=Ts_rec  MaxMissedTicks=1000  ShowMissedTicks=off  YieldWhenWaiting=off
  Subsystem : Subsystem
  Terminator : Terminator
  Terminator1 : Terminator
  Açı : Outport
  Hız : Outport  Port=2
  Akım : Outport  Port=3
  wires:
  Rate Transition3/1 -> Packet Output/3
  Rate Transition1/1 -> Packet Output/2
  Subsystem/1(Out1) -> Rate Transition5/1
  Packet Input/2 -> Subsystem/2(In2)
  Rate Transition2/1 -> Packet Output/1
  Packet Input/3 -> Subsystem/3(In3)
  Subsystem/3(Out3) -> Rate Transition6/1
  Subsystem/4(Out4) -> Rate Transition7/1
  Packet Input/1 -> Subsystem/1(In1)
  Packet Input/5 -> Subsystem/Enable
  Subsystem/2(Out2) -> Rate Transition4/1
  Rate Transition4/1 -> Açı/1
  Voltaj/1 -> Rate Transition1/1
  Constant/1 -> Rate Transition2/1
  Rate Transition7/1 -> Terminator1/1
  Constant1/1 -> Rate Transition3/1
  Rate Transition5/1 -> Terminator/1
  Packet Input/4 -> Rate Transition8/1
  Rate Transition8/1 -> Hız/1
  Packet Input/6 -> Subsystem/4(In4)
  Rate Transition6/1 -> Akım/1

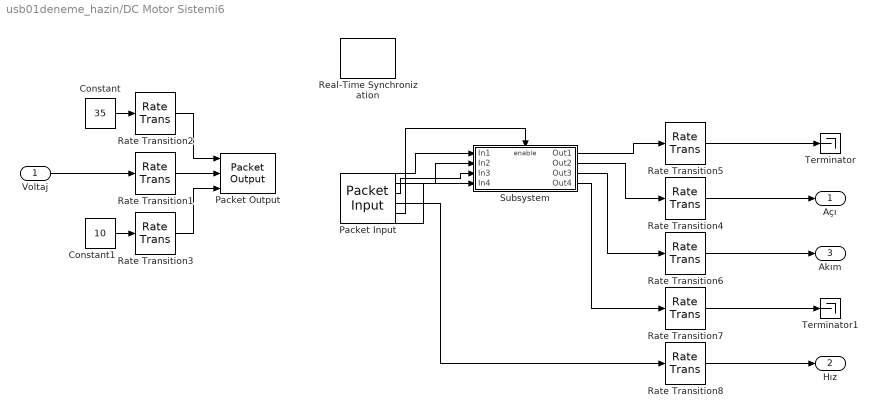
== system usb01deneme_hazin/DC Motor Sistemi6 ==
  Voltaj : Inport
  Constant : Constant  Value=35
  Constant1 : Constant  Value=10
  Packet Input : sldrtlib/Packet Input  SampleTime=Ts_rec  MaxMissedTicks=1000  ShowMissedTicks=off  YieldWhenWaiting=off  DrvName=Standard_Devices/Serial_Port  DrvAddress=4  DrvOptions=[9600 8 0 0 0 0 0 0]  PacketSize=14  DataTypes={'uint8','single','single','single','uint8'}  ShowReady=on  ShowError=off  PacketID=1  ByteOrder=1  ShowTimestamp=off
      settings: AttributesFormatString=Serial Port [4]
  Packet Output : sldrtlib/Packet Output  SampleTime=Ts_send  MaxMissedTicks=1000  ShowMissedTicks=off  YieldWhenWaiting=off  DrvName=Standard_Devices/Serial_Port  DrvAddress=4  DrvOptions=[9600 8 0 0 0 0 0 0]  PacketSize=6  DataTypes={'uint8','single','uint8'}  ShowReady=off  ShowError=off  PacketID=1  ByteOrder=1  InitialValue=[]  FinalValue=[]
      settings: AttributesFormatString=Serial Port [4]
  Rate Transition1 : RateTransition  OutPortSampleTime=Ts_send
  Rate Transition2 : RateTransition  OutPortSampleTime=Ts_send
  Rate Transition3 : RateTransition  OutPortSampleTime=Ts_send
  Rate Transition{4..8} (5 alike) : RateTransition  OutPortSampleTime=Ts_algo
  Real-Time Synchronization : sldrtlib/Real-Time Synchronization  SampleTime=Ts_rec  MaxMissedTicks=1000  ShowMissedTicks=off  YieldWhenWaiting=off
  Subsystem : Subsystem
  Terminator : Terminator
  Terminator1 : Terminator
  Açı : Outport
  Hız : Outport  Port=2
  Akım : Outport  Port=3
  wires:
  Rate Transition3/1 -> Packet Output/3
  Rate Transition1/1 -> Packet Output/2
  Subsystem/1(Out1) -> Rate Transition5/1
  Packet Input/2 -> Subsystem/2(In2)
  Rate Transition2/1 -> Packet Output/1
  Packet Input/3 -> Subsystem/3(In3)
  Subsystem/3(Out3) -> Rate Transition6/1
  Subsystem/4(Out4) -> Rate Transition7/1
  Packet Input/1 -> Subsystem/1(In1)
  Packet Input/5 -> Subsystem/Enable
  Subsystem/2(Out2) -> Rate Transition4/1
  Rate Transition4/1 -> Açı/1
  Voltaj/1 -> Rate Transition1/1
  Constant/1 -> Rate Transition2/1
  Rate Transition7/1 -> Terminator1/1
  Constant1/1 -> Rate Transition3/1
  Rate Transition5/1 -> Terminator/1
  Packet Input/4 -> Rate Transition8/1
  Rate Transition8/1 -> Hız/1
  Packet Input/6 -> Subsystem/4(In4)
  Rate Transition6/1 -> Akım/1

== system usb01deneme_hazin/PID(frequence domain emulation) ==
  e(t) : Inport
  Discrete Derivative : DiscreteZeroPole  Poles=[-1]  Gain=((2*Td)/T)  SampleTime=-1
  Discrete Integral : DiscreteZeroPole  Zeros=[-1]  Poles=[1]  Gain=(T/(2*Ti))  SampleTime=-1
  Gain : Gain  Gain=K
  Sum2 : Sum  Inputs=|+++
  u(t) : Outport
  wires:
  Sum2/1 -> u(t)/1
  Discrete Integral/1 -> Sum2/2
  Gain/1 -> Discrete Derivative/1, Discrete Integral/1, Sum2/1
  Discrete Derivative/1 -> Sum2/3
  e(t)/1 -> Gain/1

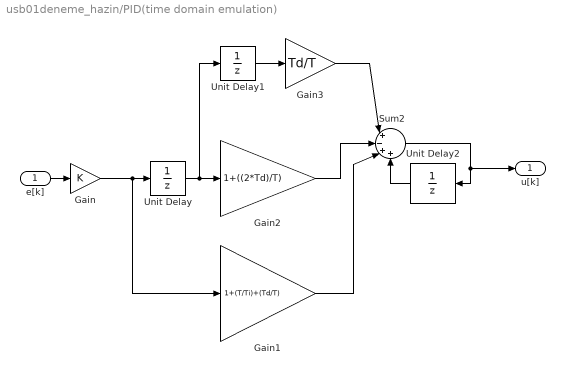
== system usb01deneme_hazin/PID(time domain emulation) ==
  e[k] : Inport
  Gain : Gain  Gain=K
  Gain1 : Gain  Gain=1+(T/Ti)+(Td/T)
  Gain2 : Gain  Gain=1+((2*Td)/T)
  Gain3 : Gain  Gain=Td/T
  Sum2 : Sum  Inputs=|+-++
  Unit Delay : UnitDelay  SampleTime=-1  HasFrameUpgradeWarning=on
  Unit Delay1 : UnitDelay  SampleTime=-1  HasFrameUpgradeWarning=on
  Unit Delay2 : UnitDelay  SampleTime=-1  HasFrameUpgradeWarning=on
  u[k] : Outport
  wires:
  Gain/1 -> Gain1/1, Unit Delay/1
  Unit Delay1/1 -> Gain3/1
  Unit Delay/1 -> Unit Delay1/1, Gain2/1
  Gain2/1 -> Sum2/2
  Gain1/1 -> Sum2/3
  Gain3/1 -> Sum2/1
  Sum2/1 -> u[k]/1, Unit Delay2/1
  Unit Delay2/1 -> Sum2/4
  e[k]/1 -> Gain/1

== system usb01deneme_hazin/numericd1 ==
  In : Inport
  Stage1 : DiscreteFilter  Tag=BlockMethodSubSystem  Numerator=[0.0360272465201760816 -0.0720544930403521633 0.0360272465201760816]  Denominator=[1 1.63889042744449531 0.782999413525199861]  InputProcessing=Columns as channels (frame based)  a0EqualsOne=on
  Stage2 : DiscreteFilter  Tag=BlockMethodSubSystem  Numerator=[0.0306469542079083335 -0.0612939084158166669 0.0306469542079083335]  Denominator=[1 1.39413928992720826 0.516727106758841703]  InputProcessing=Columns as channels (frame based)  a0EqualsOne=on
  Stage3 : DiscreteFilter  Tag=BlockMethodSubSystem  Numerator=[0.170273635614353186 -0.170273635614353186]  Denominator=[1 0.659452728771293573]  InputProcessing=Columns as channels (frame based)  a0EqualsOne=on
  Out : Outport
  wires:
  In/1 -> Stage1/1
  Stage1/1 -> Stage2/1
  Stage2/1 -> Stage3/1
  Stage3/1 -> Out/1

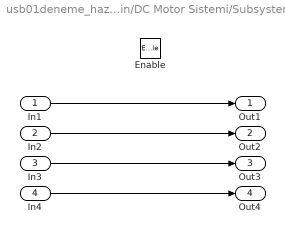
== system usb01deneme_hazin/DC Motor Sistemi/Subsystem ==
  In1 : Inport
  In2 : Inport  Port=2
  In3 : Inport  Port=3
  In4 : Inport  Port=4
  Enable : EnablePort
  Out1 : Outport
  Out2 : Outport  Port=2
  Out3 : Outport  Port=3
  Out4 : Outport  Port=4
  wires:
  In1/1 -> Out1/1
  In2/1 -> Out2/1
  In3/1 -> Out3/1
  In4/1 -> Out4/1

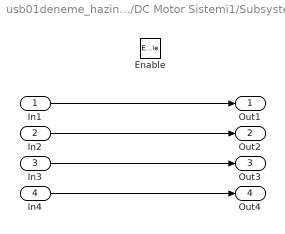
== system usb01deneme_hazin/DC Motor Sistemi1/Subsystem ==
  In1 : Inport
  In2 : Inport  Port=2
  In3 : Inport  Port=3
  In4 : Inport  Port=4
  Enable : EnablePort
  Out1 : Outport
  Out2 : Outport  Port=2
  Out3 : Outport  Port=3
  Out4 : Outport  Port=4
  wires:
  In1/1 -> Out1/1
  In2/1 -> Out2/1
  In3/1 -> Out3/1
  In4/1 -> Out4/1

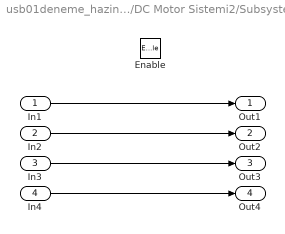
== system usb01deneme_hazin/DC Motor Sistemi2/Subsystem ==
  In1 : Inport
  In2 : Inport  Port=2
  In3 : Inport  Port=3
  In4 : Inport  Port=4
  Enable : EnablePort
  Out1 : Outport
  Out2 : Outport  Port=2
  Out3 : Outport  Port=3
  Out4 : Outport  Port=4
  wires:
  In1/1 -> Out1/1
  In2/1 -> Out2/1
  In3/1 -> Out3/1
  In4/1 -> Out4/1

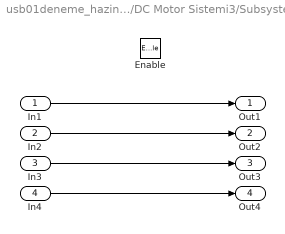
== system usb01deneme_hazin/DC Motor Sistemi3/Subsystem ==
  In1 : Inport
  In2 : Inport  Port=2
  In3 : Inport  Port=3
  In4 : Inport  Port=4
  Enable : EnablePort
  Out1 : Outport
  Out2 : Outport  Port=2
  Out3 : Outport  Port=3
  Out4 : Outport  Port=4
  wires:
  In1/1 -> Out1/1
  In2/1 -> Out2/1
  In3/1 -> Out3/1
  In4/1 -> Out4/1

== system usb01deneme_hazin/DC Motor Sistemi4/Subsystem ==
  In1 : Inport
  In2 : Inport  Port=2
  In3 : Inport  Port=3
  In4 : Inport  Port=4
  Enable : EnablePort
  Out1 : Outport
  Out2 : Outport  Port=2
  Out3 : Outport  Port=3
  Out4 : Outport  Port=4
  wires:
  In1/1 -> Out1/1
  In2/1 -> Out2/1
  In3/1 -> Out3/1
  In4/1 -> Out4/1

== system usb01deneme_hazin/DC Motor Sistemi6/Subsystem ==
  In1 : Inport
  In2 : Inport  Port=2
  In3 : Inport  Port=3
  In4 : Inport  Port=4
  Enable : EnablePort
  Out1 : Outport
  Out2 : Outport  Port=2
  Out3 : Outport  Port=3
  Out4 : Outport  Port=4
  wires:
  In1/1 -> Out1/1
  In2/1 -> Out2/1
  In3/1 -> Out3/1
  In4/1 -> Out4/1

== matlab function usb01deneme_hazin/MATLAB Function ==
  data: e input; norme output
function norme = fcn(e)
%#codegen

norme = norm(e)^2;

== matlab function usb01deneme_hazin/MATLAB Function2 ==
  data: e input; norme output
function norme = fcn(e)
%#codegen

norme = norm(e)^2;

== matlab function usb01deneme_hazin/MATLAB Function1 ==
  data: e input; norme output
function norme = fcn(e)
%#codegen

norme = norm(e)^2;
